simulink model "DaVinci_Simul_IK"  (R2023a)
settings: Solver=VariableStepAuto  StartTime=0.0  StopTime=inf  RelTol=1e-3  EnableMultiTasking=on
libraries: vrlib x7, DaVinci_Lib x2
settings Model: Creator=jorgemartins  LastModifiedBy=afons
settings SolverCC: AlgebraicLoopSolver=TrustRegion
settings DataIOCC: LimitDataPoints=on  ReturnWorkspaceOutputs=off
settings OptimizationCC: LifeSpan=inf
settings DebuggingCC: UnconnectedInputMsg=warning  UnconnectedOutputMsg=warning  UnconnectedLineMsg=warning  AllowSymbolicDim=off  SFUnexpectedBacktrackingDiag=warning  SFNoUnconditionalDefaultTransitionDiag=warning  SFExecutionAtInitializationDiag=none  ArithmeticOperatorsInVariantConditions=warning
settings ModelReferenceCC: EnableRefExpFcnMdlSchedulingChecks=on  PropagateSignalLabelsOutOfModel=off
settings SFSimCC: SimUseLocalCustomCode=off  CustomCodeUndefinedFunction=UseInterfaceOnly
settings RTWCC: RTWUseLocalCustomCode=off
settings CodeAppCC: StateflowObjectComments=on
settings GRTTargetCC: TargetLangStandard=C89/C90 (ANSI)
settings ConfigComp: CovMetricSettings=dw  CovSaveCumulativeToWorkspaceVar=on  CovSaveSingleToWorkspaceVar=on  CovExternalEMLEnable=off

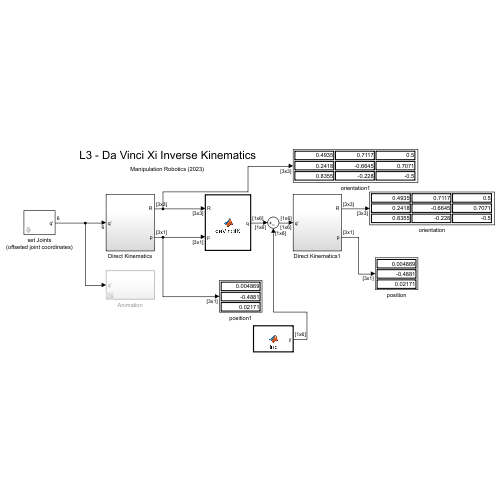
[thumbnail: Simulink's stored preview of the top-level diagram]
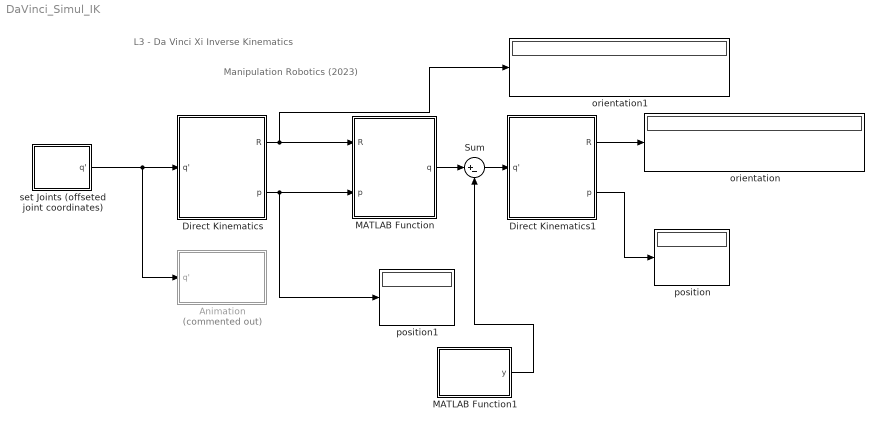
== system DaVinci_Simul_IK ==
  note: Manipulation Robotics (2023)
  note: L3 - Da Vinci Xi Inverse Kinematics
  Animation : Subsystem  Commented=on
  Direct Kinematics : Subsystem
  Direct Kinematics1 : Subsystem
  MATLAB Function : MATLAB Function  TreatAsAtomicUnit=on
  MATLAB Function1 : MATLAB Function  TreatAsAtomicUnit=on
  Sum : Sum  Inputs=|+-
  orientation : Display
  orientation1 : Display
  position : Display
  position1 : Display
  set Joints (offseted joint coordinates) : Subsystem  mask{q1=90, q2=0, q3=0.5, q4=-45, q5=135, q6=70}
  wires:
  set Joints (offseted joint coordinates)/1(q') -> Animation/1(q'), Direct Kinematics/1(q')
  Direct Kinematics/2(p) -> position1/1, MATLAB Function/2(p)
  Direct Kinematics/1(R) -> orientation1/1, MATLAB Function/1(R)
  Direct Kinematics1/1(R) -> orientation/1
  Direct Kinematics1/2(p) -> position/1
  Sum/1 -> Direct Kinematics1/1(q')
  MATLAB Function/1(q) -> Sum/1
  MATLAB Function1/1(y) -> Sum/2

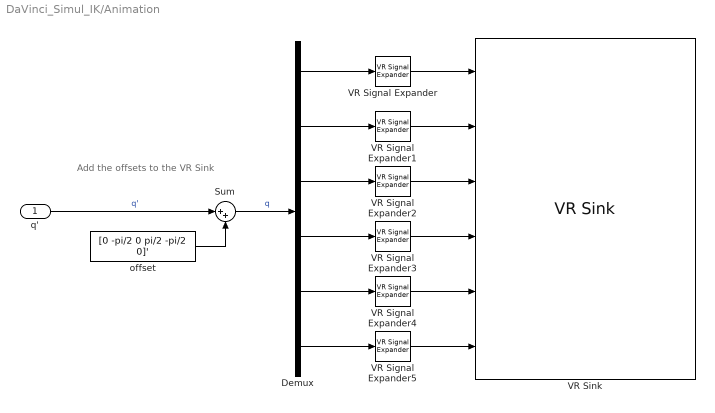
== system DaVinci_Simul_IK/Animation ==
  note: Add the offsets to the VR Sink
  q' : Inport
  Demux : Demux  Outputs=6
  Sum : Sum  Inputs=|++
  VR Signal Expander{,1,3..5} (5 alike) : vrlib/VR Signal Expander  outwidth=4  outidx=[4]
  VR Signal Expander2 : vrlib/VR Signal Expander  outwidth=3  outidx=[3]
  VR Sink : vrlib/VR Sink  InstantiateOnLoad=on  SampleTime=-1  ViewEnable=on  RemoteChange=off  RemoteView=off  FieldsWritten=Jt1_DH_dv.rotation.4.1.1.double#Jt2_DH_dv.rotation.4.1.1.double#Jt3_DH_dv.translation.3.1.1.double#Jt4_DH_dv.rotation.4.1.1.double#Jt5_DH_dv.rotation.4.1.1.double#Jt6_DH_dv.rotation.4.1.1.double  WorldFileName=DaVinciFrames.wrl  WorldDescription=Da Vinci Frames  AutoView=on  VideoDimensions=[]  AllowVariableSize=off
  offset : Constant  Value=[0 -pi/2 0 pi/2 -pi/2 0]'  VectorParams1D=off
  wires:
  VR Signal Expander2/1 -> VR Sink/3
  offset/1 -> Sum/2
  VR Signal Expander1/1 -> VR Sink/2
  q'/1 -> Sum/1  "q'"
  Sum/1 -> Demux/1  "q"
  Demux/3 -> VR Signal Expander2/1
  Demux/6 -> VR Signal Expander5/1
  VR Signal Expander3/1 -> VR Sink/4
  Demux/1 -> VR Signal Expander/1
  Demux/2 -> VR Signal Expander1/1
  VR Signal Expander4/1 -> VR Sink/5
  Demux/4 -> VR Signal Expander3/1
  Demux/5 -> VR Signal Expander4/1
  VR Signal Expander5/1 -> VR Sink/6
  VR Signal Expander/1 -> VR Sink/1

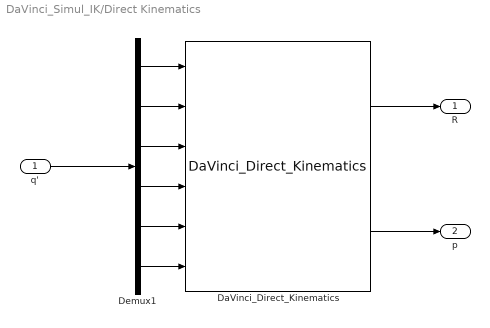
== system DaVinci_Simul_IK/Direct Kinematics ==
  q' : Inport
  DaVinci_Direct_Kinematics : DaVinci_Lib/DaVinci_Direct_Kinematics  SystemSampleTime=-1  VariantActivationTime=update diagram  Latency=0  AutoFrameSizeCalculation=off
  Demux1 : Demux  Outputs=6
  R : Outport
  p : Outport  Port=2
  wires:
  DaVinci_Direct_Kinematics/1 -> R/1
  DaVinci_Direct_Kinematics/2 -> p/1
  q'/1 -> Demux1/1
  Demux1/6 -> DaVinci_Direct_Kinematics/6
  Demux1/1 -> DaVinci_Direct_Kinematics/1
  Demux1/4 -> DaVinci_Direct_Kinematics/4
  Demux1/2 -> DaVinci_Direct_Kinematics/2
  Demux1/5 -> DaVinci_Direct_Kinematics/5
  Demux1/3 -> DaVinci_Direct_Kinematics/3

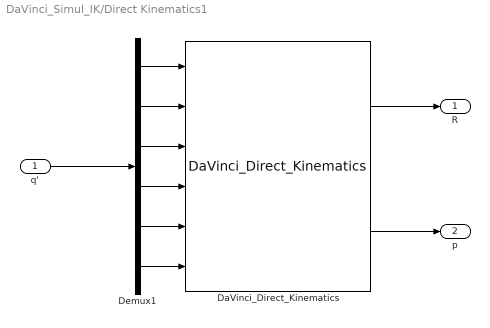
== system DaVinci_Simul_IK/Direct Kinematics1 ==
  q' : Inport
  DaVinci_Direct_Kinematics : DaVinci_Lib/DaVinci_Direct_Kinematics  SystemSampleTime=-1  VariantActivationTime=update diagram  Latency=0  AutoFrameSizeCalculation=off
  Demux1 : Demux  Outputs=6
  R : Outport
  p : Outport  Port=2
  wires:
  DaVinci_Direct_Kinematics/1 -> R/1
  DaVinci_Direct_Kinematics/2 -> p/1
  q'/1 -> Demux1/1
  Demux1/6 -> DaVinci_Direct_Kinematics/6
  Demux1/1 -> DaVinci_Direct_Kinematics/1
  Demux1/4 -> DaVinci_Direct_Kinematics/4
  Demux1/2 -> DaVinci_Direct_Kinematics/2
  Demux1/5 -> DaVinci_Direct_Kinematics/5
  Demux1/3 -> DaVinci_Direct_Kinematics/3

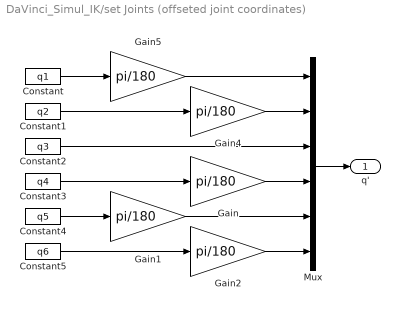
== system DaVinci_Simul_IK/set Joints (offseted joint coordinates) ==
  Constant : Constant  Value=q1
  Constant1 : Constant  Value=q2
  Constant2 : Constant  Value=q3
  Constant3 : Constant  Value=q4
  Constant4 : Constant  Value=q5
  Constant5 : Constant  Value=q6
  Gain{,1..2,4..5} (5 alike) : Gain  Gain=pi/180
  Mux : Mux  Inputs=6
  q' : Outport
  wires:
  Gain2/1 -> Mux/6
  Constant1/1 -> Gain4/1
  Constant3/1 -> Gain/1
  Constant5/1 -> Gain2/1
  Mux/1 -> q'/1
  Gain5/1 -> Mux/1
  Gain/1 -> Mux/4
  Gain1/1 -> Mux/5
  Gain4/1 -> Mux/2
  Constant/1 -> Gain5/1
  Constant2/1 -> Mux/3
  Constant4/1 -> Gain1/1

== matlab function DaVinci_Simul_IK/MATLAB Function ==
  data: R input; q output; p input
function q  = daVinciIK(R, p)
% IKin Calculations for DaVinci Robot
% q = [qx qy qz]

ii = [1 ; 0 ; 0];
jj = [0 ; 1 ; 0];
kk = [0 ; 0 ; 1];
a5 = .010;
a6 = .020;

x6 = R * ii;
y6 = R * jj;
z6 = R * kk;
p5 = p - a6 * x6;
z5 = z6;

z4 = cross(p5, z5) / norm(cross(p5, z5));
x5 = cross(z5, z4);
p3 = p5 - a5 * x5;

theta1 = atan2(-jj.' * p3, -ii.' * p3);
R1 = [cos(theta1) 0 -sin(theta1) ; sin(theta1) 0 cos(theta1) ; 0 -1 0];
x1 = R1 * ii;
y1 = R1 * jj;
z1 = cross(x1, y1);


theta2 = -atan2(-x1.' * p3, -y1.' * p3);
d3 = norm(p3);
z3 = p3 / norm(p3);
x4 = cross(z4, z3);
theta5 = -atan2(z5.' * x4, x5.' * x4);
y5 = cross(z5, x5);



theta6 = atan2(y5.' * x6, x5.' * x6);
R3 = [cos(theta1)*cos(theta2) , -sin(theta1) , cos(theta1)*sin(theta2) ; 
    sin(theta1) * cos(theta2) , cos(theta1) , sin(theta1) * sin(theta2) ; 
    -sin(theta2) , 0 , cos(theta2)];
x3 = R3 * ii;
y3 = R3 * jj;
theta4 = atan2(y3.' * x4, x3.' * x4);

q = [theta1 theta2 d3 theta4 theta5 theta6]

end

== matlab function DaVinci_Simul_IK/MATLAB Function1 ==
  data: y output
function y = fnc
%#codegen


y = [0 , -pi/2 , 0 , pi/2 , -pi/2 , 0];

end
